simulink model "STR_roirac"  (R2013a)
settings: Solver=ode5  SolverMode=SingleTasking  StartTime=0.0  StopTime=20  FixedStep=0.005  RelTol=1e-3
settings Model: CovMetricSettings=dwe  CovHtmlReporting=off  covSaveCumulativeToWorkspaceVar=off  CovSaveSingleToWorkspaceVar=off  CovExternalEMLEnable=on  Creator=Administrator  LastModifiedBy=Administrator
settings DataIOCC: LimitDataPoints=off  SaveFormat=StructureWithTime
settings DebuggingCC: UnderspecifiedInitializationDetection=Simplified  MergeDetectMultiDrivingBlocksExec=error  SolverPrmCheckMsg=none  FrameProcessingCompatibilityMsg=error  StateNameClashWarn=none  SFUnexpectedBacktrackingDiag=error  SFNoUnconditionalDefaultTransitionDiag=error
settings HardwareCC: ProdBitPerPointer=64  ProdLargestAtomicFloat=Float  ProdIntDivRoundTo=Zero  ProdEndianess=LittleEndian  ProdHWDeviceType=Specified
settings ModelReferenceCC: PropagateSignalLabelsOutOfModel=on
settings GRTTargetCC: CodeReplacementLibrary=C99 (ISO)  GeneratePreprocessorConditionals=Use local settings

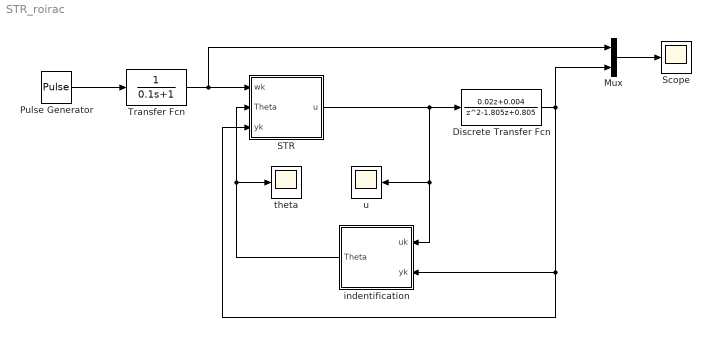
== system STR_roirac ==
  Discrete Transfer Fcn : DiscreteTransferFcn  Numerator=[0.02 0.004]  Denominator=[1 -1.805 0.805]
  Mux : Mux  Inputs=2
  Pulse Generator : DiscretePulseGenerator  PulseType=Time based  Period=4  PulseWidth=50
  STR : Subsystem
  Scope : Scope
      settings: TimeRange=auto  MaxDataPoints=5000  SaveToWorkspace=off  SaveName=ScopeData  YMin=-0.125  YMax=1.125  SampleTime=-1  DataFormat=Array
  Transfer Fcn : TransferFcn  Denominator=[0.1 1]
  indentification : Subsystem
  theta : Scope
      settings: TimeRange=auto  MaxDataPoints=5000  SaveToWorkspace=off  YMin=-10  YMax=10  SampleTime=-1
  u : Scope
      settings: TimeRange=auto  LimitDataPoints=on  MaxDataPoints=5000  SaveToWorkspace=off  SaveName=ScopeData2  YMin=-10  YMax=10  SampleTime=-1  DataFormat=Array
  wires:
  Pulse Generator/1 -> Transfer Fcn/1
  Transfer Fcn/1 -> STR/1(wk), Mux/1
  STR/1(u) -> Discrete Transfer Fcn/1, indentification/1(uk), u/1
  Mux/1 -> Scope/1
  Discrete Transfer Fcn/1 -> indentification/2(yk), STR/3(yk), Mux/2
  indentification/1(Theta) -> theta/1, STR/2(Theta)

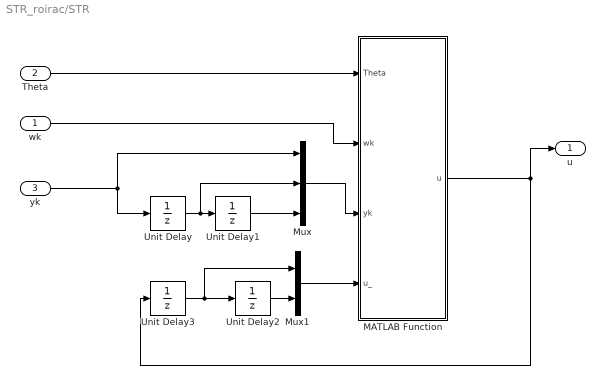
== system STR_roirac/STR ==
  wk : Inport  PortDimensions=1
  Theta : Inport  Port=2  PortDimensions=4
  yk : Inport  Port=3  PortDimensions=1
  MATLAB Function : MATLAB Function  TreatAsAtomicUnit=on
      settings: PermitHierarchicalResolution=ParametersOnly
  Mux : Mux  Inputs=3
  Mux1 : Mux  Inputs=2
  Unit Delay{,1..3} (4 alike) : UnitDelay  SampleTime=-1
  u : Outport  PortDimensions=1
  wires:
  Theta/1 -> MATLAB Function/1(Theta)
  wk/1 -> MATLAB Function/2(wk)
  Unit Delay/1 -> Mux/2, Unit Delay1/1
  Unit Delay1/1 -> Mux/3
  Mux/1 -> MATLAB Function/3(yk)
  MATLAB Function/1(u) -> Unit Delay3/1, u/1
  Unit Delay3/1 -> Mux1/1, Unit Delay2/1
  Unit Delay2/1 -> Mux1/2
  Mux1/1 -> MATLAB Function/4(u_)
  yk/1 -> Unit Delay/1, Mux/1

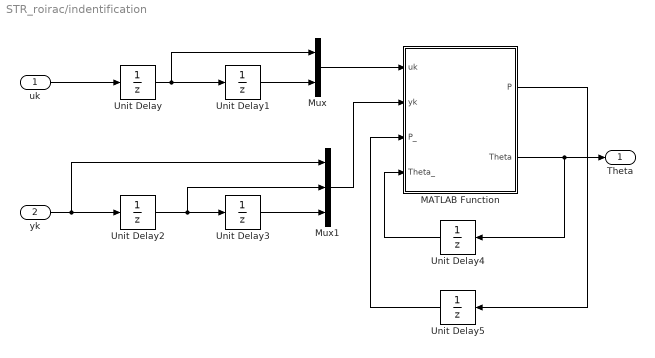
== system STR_roirac/indentification ==
  uk : Inport  PortDimensions=1
  yk : Inport  Port=2  PortDimensions=1
  MATLAB Function : MATLAB Function  TreatAsAtomicUnit=on
      settings: PermitHierarchicalResolution=ParametersOnly
  Mux : Mux  Inputs=2
  Mux1 : Mux  Inputs=3
  Unit Delay{,1..3} (4 alike) : UnitDelay  SampleTime=-1
  Unit Delay4 : UnitDelay  InitialCondition=rand(4,1)  SampleTime=-1
  Unit Delay5 : UnitDelay  InitialCondition=1e5*eye(4)  SampleTime=-1
  Theta : Outport  PortDimensions=4
  wires:
  uk/1 -> Unit Delay/1
  Unit Delay/1 -> Mux/1, Unit Delay1/1
  Unit Delay1/1 -> Mux/2
  Mux/1 -> MATLAB Function/1(uk)
  Unit Delay3/1 -> Mux1/3
  Unit Delay2/1 -> Mux1/2, Unit Delay3/1
  yk/1 -> Mux1/1, Unit Delay2/1
  Mux1/1 -> MATLAB Function/2(yk)
  MATLAB Function/2(Theta) -> Unit Delay4/1, Theta/1
  Unit Delay4/1 -> MATLAB Function/4(Theta_)
  MATLAB Function/1(P) -> Unit Delay5/1
  Unit Delay5/1 -> MATLAB Function/3(P_)

== matlab function STR_roirac/STR/MATLAB Function ==
  data: Theta input; u output; wk input; yk input; u_ input

% Ham tinh thong so bo dieu khien theo pp dat cuc lien tuc
function u = STR_pp1(Theta,wk,yk,u_)
alp = 0.001;
bet = 0.003;
% Gan lai thong so de thuan tien viec tinh toan
a1 = Theta(1);
a2 = Theta(2);
b1 = Theta(3);
b2 = Theta(4);
% Tinh thong so bo dieu khien
x1=-4*alp+1-a1;
x2=6*alp^2+bet^2+a1-a2;
x3=2*alp*(2*alp^2+bet^2)-a2;
x4=alp^2*(alp^2+bet^2);
r1=(b1+b2)*(a1*b1*b2-a2*b1^2-b2^2);
r2=a1*b2*(b1*(x2-x3+x4)-b2*x1);
r3=a2*b1*(b2*x1-b1*(x2-x3+x4));
r4=(b1+b2)*(b1*x4+b2*(x3-x4));
r5=b1*(b1^2*x4+b1*b2*x3+b2^2*x2)-b2^3*x1;
r6=b1^2*(a2*x3+a1*x4-a2*x4);
r7=b2*(b1*(a1*x4+a2*x2-x4)-b2*(a2*x1+x4));
r0=(x1+x2-x3+x4)/(b1+b2);
p1=(r5-r1)/r1;
p2=-r5/r1;
q0=r0-(r2+r3+r4)/r1;
q1=(r2+r3+r4-r6-r7)/r1;
q2=(r6+r7)/r1;
% Luat dieu khien
u = r0*wk - q0*yk(1) - q1*yk(2) - q2*yk(3) - p1*u_(1) - p2*u_(2);

== matlab function STR_roirac/indentification/MATLAB Function ==
  data: uk input; P output; yk input; P_ input; Theta_ input; Theta output
% Ham nhan dang thong so doi tuong
function [P,Theta] = Uocluong(uk,yk,P_,Theta_)
lamda = 0.96;
PHI = [-yk(2); -yk(3); uk(1); uk(2)];
e = yk(1) - PHI'*Theta_;
L = P_*PHI / (lamda + PHI'*P_*PHI);
P = 1/lamda*(P_ - P_*PHI*PHI'*P_ /(lamda + PHI'*P_*PHI));
Theta = Theta_ + L*e;
